simulink model "Aero_Generic"  (R2016b)
settings: Solver=VariableStepAuto  StartTime=0.0  StopTime=10.0  RelTol=1e-3
values from neighbouring files (symbols this model uses):
  AC =     [UAV_modelconfig.mat]
libraries: OpenFlightUtilLib x3
settings Model: Creator=UAVLAB  LastModifiedBy=rega0051

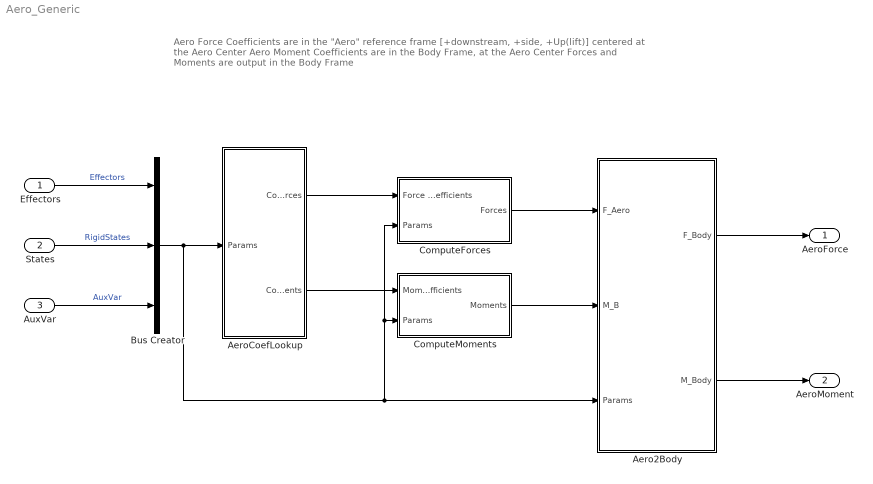
== system Aero_Generic ==
  note: Aero Force Coefficients are in the "Aero" reference frame [+downstream, +side, +Up(lift)] centered at the Aero Center
      | Aero Moment Coefficients are in the Body Frame, at the Aero Center
      |
      | Forces and Moments are output in the Body Frame
  Effectors : Inport  OutDataTypeStr=Bus: Effectors
  States : Inport  Port=2  OutDataTypeStr=Bus: RigidStates
  AuxVar : Inport  Port=3  OutDataTypeStr=Bus: AuxVar
  Aero2Body : Subsystem
  AeroCoefLookup : Subsystem
  Bus Creator : BusCreator  Inputs=3
  ComputeForces : Subsystem
  ComputeMoments : Subsystem
  AeroForce : Outport
  AeroMoment : Outport  Port=2
  wires:
  States/1 -> Bus Creator/2  "RigidStates"
  AuxVar/1 -> Bus Creator/3  "AuxVar"
  Effectors/1 -> Bus Creator/1  "Effectors"
  Bus Creator/1 -> Aero2Body/3(Params), ComputeForces/2(Params), ComputeMoments/2(Params), AeroCoefLookup/1(Params)
  ComputeForces/1(Forces) -> Aero2Body/1(F_Aero)
  ComputeMoments/1(Moments) -> Aero2Body/2(M_B)
  Aero2Body/1(F_Body) -> AeroForce/1
  Aero2Body/2(M_Body) -> AeroMoment/1
  AeroCoefLookup/1(CoefForces) -> ComputeForces/1(Force Coefficients)
  AeroCoefLookup/2(CoefMoments) -> ComputeMoments/1(Moment Coefficients)

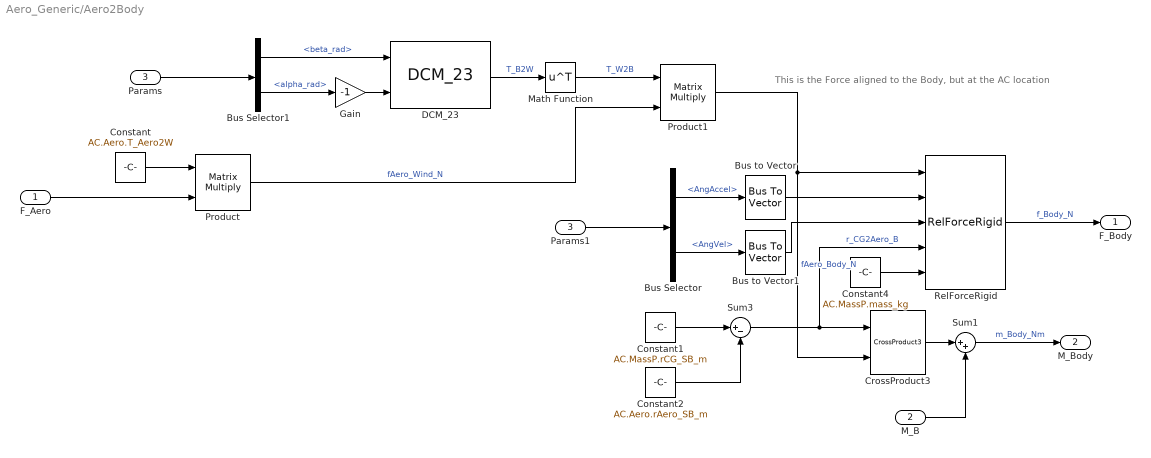
== system Aero_Generic/Aero2Body ==
  note: This is the Force aligned to the Body, but at the AC location
  F_Aero : Inport
  M_B : Inport  Port=2
  Params : Inport  Port=3
  Bus Selector : BusSelector  OutputSignals=RigidStates.AngAccel,RigidStates.AngVel
  Bus Selector1 : BusSelector  OutputSignals=AuxVar.WindAxesParams.beta_rad,AuxVar.WindAxesParams.alpha_rad
  Bus to Vector : BusToVector
  Bus to Vector1 : BusToVector
  Constant : Constant  Value=AC.Aero.T_Aero2W
      settings: AttributesFormatString=%<Value>
  Constant1 : Constant  Value=AC.MassP.rCG_SB_m
      settings: AttributesFormatString=%<Value>
  Constant2 : Constant  Value=AC.Aero.rAero_SB_m
      settings: AttributesFormatString=%<Value>
  Constant4 : Constant  Value=AC.MassP.mass_kg
      settings: AttributesFormatString=%<Value>
  CrossProduct3 : OpenFlightUtilLib/Math/CrossProduct3
  DCM_23 : OpenFlightUtilLib/Transformations/DCM_23
  Gain : Gain  Gain=-1
  Math Function : Math  Operator=transpose  SaturateOnIntegerOverflow=on
  Params1 : InportShadow  Port=3
  Product : Product  Multiplication=Matrix(*)  RndMeth=Zero
  Product1 : Product  Multiplication=Matrix(*)  RndMeth=Zero
  RelForceRigid : OpenFlightUtilLib/Kinematics and Dynamics/RelForceRigid
  Sum1 : Sum  Inputs=|++  SaturateOnIntegerOverflow=on
  Sum3 : Sum  Inputs=|+-  SaturateOnIntegerOverflow=on
  F_Body : Outport
  M_Body : Outport  Port=2
  wires:
  Constant1/1 -> Sum3/1
  Constant2/1 -> Sum3/2
  Bus Selector/1 -> Bus to Vector/1  "<AngAccel>"
  Bus to Vector/1 -> RelForceRigid/2
  Bus to Vector1/1 -> RelForceRigid/3
  Bus Selector/2 -> Bus to Vector1/1  "<AngVel>"
  F_Aero/1 -> Product/2
  Constant/1 -> Product/1
  Params/1 -> Bus Selector1/1
  Math Function/1 -> Product1/1  "T_W2B"
  DCM_23/1 -> Math Function/1  "T_B2W"
  Product/1 -> Product1/2  "fAero_Wind_N"
  Product1/1 -> CrossProduct3/2, RelForceRigid/1  "fAero_Body_N"
  Sum3/1 -> RelForceRigid/4, CrossProduct3/1  "r_CG2Aero_B"
  Params1/1 -> Bus Selector/1
  RelForceRigid/1 -> F_Body/1  "f_Body_N"
  M_B/1 -> Sum1/2
  CrossProduct3/1 -> Sum1/1
  Sum1/1 -> M_Body/1  "m_Body_Nm"
  Constant4/1 -> RelForceRigid/5
  Bus Selector1/1 -> DCM_23/1  "<beta_rad>"
  Bus Selector1/2 -> Gain/1  "<alpha_rad>"
  Gain/1 -> DCM_23/2

== system Aero_Generic/AeroCoefLookup ==
  Params : Inport
  DragCoefficient : Subsystem
  Lift Coefficient : Subsystem
  Mux : Mux  Inputs=3
  Mux1 : Mux  Inputs=3
  PitchMomentCoefficient : Subsystem
  RollMomentCoefficient : Subsystem
  SideForceCoefficient : Subsystem
  YawMomentCoefficient : Subsystem
  CoefForces : Outport
  CoefMoments : Outport  Port=2
  wires:
  Mux1/1 -> CoefMoments/1  "coefMom_B"
  SideForceCoefficient/1(CY) -> Mux/2
  PitchMomentCoefficient/1(Cm) -> Mux1/2
  Mux/1 -> CoefForces/1  "coefF_Aero"
  RollMomentCoefficient/1(Cl) -> Mux1/1
  Lift Coefficient/1(CL) -> DragCoefficient/2(CL), Mux/3
  YawMomentCoefficient/1(Cn) -> Mux1/3
  DragCoefficient/1(CD) -> Mux/1
  Params/1 -> YawMomentCoefficient/1(Params), PitchMomentCoefficient/1(Params), RollMomentCoefficient/1(Params), Lift Coefficient/1(Params), SideForceCoefficient/1(Params), DragCoefficient/1(Params)

== system Aero_Generic/ComputeForces ==
  Force Coefficients : Inport
  Params : Inport  Port=2
  Bus Selector : BusSelector  OutputSignals=AuxVar.qBar_Pa
  Demux3 : Demux  Outputs=3
  Gain2 : Gain  Gain=AC.Geometry.S  SaturateOnIntegerOverflow=on  OutDataTypeStr=Inherit: Same as input  ParamDataTypeStr=Inherit: Same as input
      settings: AttributesFormatString=%<Gain>
  Mux1 : Mux  Inputs=3
  Product6 : Product  SaturateOnIntegerOverflow=on  InputSameDT=on  OutDataTypeStr=Inherit: Same as first input
  Product7 : Product  SaturateOnIntegerOverflow=on  InputSameDT=on  OutDataTypeStr=Inherit: Same as first input
  Product8 : Product  SaturateOnIntegerOverflow=on  InputSameDT=on  OutDataTypeStr=Inherit: Same as first input
  Forces : Outport
  wires:
  Product6/1 -> Mux1/1  "fD_N"
  Product8/1 -> Mux1/3  "fL_N"
  Product7/1 -> Mux1/2  "fY_N"
  Mux1/1 -> Forces/1  "fAero_N"
  Demux3/2 -> Product7/1  "cY"
  Demux3/1 -> Product6/1  "cD"
  Demux3/3 -> Product8/1  "cL"
  Force Coefficients/1 -> Demux3/1
  Gain2/1 -> Product6/2, Product7/2, Product8/2
  Bus Selector/1 -> Gain2/1  "<qBar_Pa>"
  Params/1 -> Bus Selector/1

== system Aero_Generic/ComputeMoments ==
  Moment Coefficients : Inport
  Params : Inport  Port=2
  Bus Selector : BusSelector  OutputSignals=AuxVar.qBar_Pa
  Demux3 : Demux  Outputs=3
  Gain1 : Gain  Gain=AC.Geometry.b  SaturateOnIntegerOverflow=on  OutDataTypeStr=Inherit: Same as input  ParamDataTypeStr=Inherit: Same as input
      settings: AttributesFormatString=%<Gain>
  Gain2 : Gain  Gain=AC.Geometry.S  SaturateOnIntegerOverflow=on  OutDataTypeStr=Inherit: Same as input  ParamDataTypeStr=Inherit: Same as input
      settings: AttributesFormatString=%<Gain>
  Gain3 : Gain  Gain=AC.Geometry.b  SaturateOnIntegerOverflow=on  OutDataTypeStr=Inherit: Same as input  ParamDataTypeStr=Inherit: Same as input
      settings: AttributesFormatString=%<Gain>
  Gain4 : Gain  Gain=AC.Geometry.c  SaturateOnIntegerOverflow=on  OutDataTypeStr=Inherit: Same as input  ParamDataTypeStr=Inherit: Same as input
      settings: AttributesFormatString=%<Gain>
  Mux1 : Mux  Inputs=3
  Product6 : Product  SaturateOnIntegerOverflow=on  InputSameDT=on  OutDataTypeStr=Inherit: Same as first input
  Product7 : Product  SaturateOnIntegerOverflow=on  InputSameDT=on  OutDataTypeStr=Inherit: Same as first input
  Product8 : Product  SaturateOnIntegerOverflow=on  InputSameDT=on  OutDataTypeStr=Inherit: Same as first input
  Moments : Outport
  wires:
  Product6/1 -> Mux1/1  "mL_Nm"
  Product8/1 -> Mux1/3  "mN_Nm"
  Moment Coefficients/1 -> Demux3/1
  Product7/1 -> Mux1/2  "mM_Nm"
  Gain3/1 -> Product8/2
  Mux1/1 -> Moments/1  "mAero_Nm"
  Gain1/1 -> Product6/2
  Gain2/1 -> Gain1/1, Gain4/1, Gain3/1
  Demux3/2 -> Product7/1  "Cm"
  Gain4/1 -> Product7/2
  Demux3/1 -> Product6/1  "Cl"
  Demux3/3 -> Product8/1  "Cn"
  Bus Selector/1 -> Gain2/1  "<qBar_Pa>"
  Params/1 -> Bus Selector/1

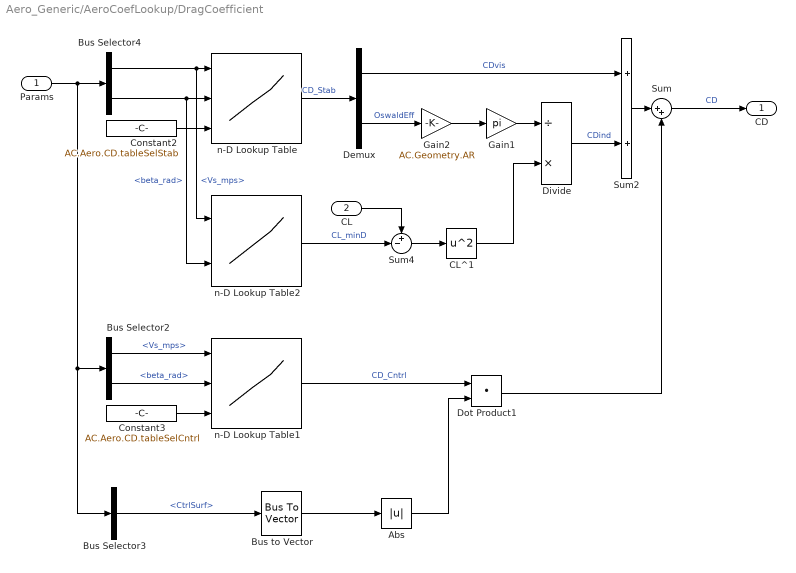
== system Aero_Generic/AeroCoefLookup/DragCoefficient ==
  Params : Inport
  CL : Inport  Port=2
  Abs : Abs
  Bus Selector2 : BusSelector  OutputSignals=AuxVar.WindAxesParams.Vs_mps,AuxVar.WindAxesParams.beta_rad
  Bus Selector3 : BusSelector  OutputSignals=Effectors.CtrlSurf
  Bus Selector4 : BusSelector  OutputSignals=AuxVar.WindAxesParams.Vs_mps,AuxVar.WindAxesParams.beta_rad
  Bus to Vector : BusToVector
  CL^1 : Math  Operator=square  SaturateOnIntegerOverflow=on
  Constant2 : Constant  Value=AC.Aero.CD.tableSelStab
      settings: AttributesFormatString=%<Value>
  Constant3 : Constant  Value=AC.Aero.CD.tableSelCntrl
      settings: AttributesFormatString=%<Value>
  Demux : Demux  Outputs=length(AC.Aero.CD.tableSelStab)
  Divide : Product  Inputs=/*
  Dot Product1 : DotProduct  InputSameDT=on  OutDataTypeStr=Inherit: Inherit via internal rule
  Gain1 : Gain  Gain=pi  SaturateOnIntegerOverflow=on  OutDataTypeStr=Inherit: Same as input  ParamDataTypeStr=Inherit: Same as input
      settings: AttributesFormatString=%<Gain>
  Gain2 : Gain  Gain=AC.Geometry.AR  SaturateOnIntegerOverflow=on  OutDataTypeStr=Inherit: Same as input  ParamDataTypeStr=Inherit: Same as input
      settings: AttributesFormatString=%<Gain>
  Sum : Sum  Inputs=|++
  Sum2 : Sum  SaturateOnIntegerOverflow=on  InputSameDT=on  OutDataTypeStr=Inherit: Same as first input
  Sum4 : Sum  Inputs=+-|  SaturateOnIntegerOverflow=on  InputSameDT=on  OutDataTypeStr=Inherit: Same as first input
  n-D Lookup Table : Lookup_n-D  NumberOfTableDimensions=3  BreakpointsForDimension1=AC.Aero.breakPts{1}  BreakpointsForDimension2=AC.Aero.breakPts{2}  BreakpointsForDimension3=AC.Aero.CD.tableSelStab  Table=AC.Aero.CD.tableStab  InternalRulePriority=Speed  RndMeth=Simplest  InputSameDT=on
      settings: AttributesFormatString=%<Table>
  n-D Lookup Table1 : Lookup_n-D  NumberOfTableDimensions=3  BreakpointsForDimension1=AC.Aero.breakPts{1}  BreakpointsForDimension2=AC.Aero.breakPts{2}  BreakpointsForDimension3=AC.Aero.CD.tableSelCntrl  Table=AC.Aero.CD.tableCntrl  InternalRulePriority=Speed  RndMeth=Simplest  InputSameDT=on
      settings: AttributesFormatString=%<Table>
  n-D Lookup Table2 : Lookup_n-D  BreakpointsForDimension1=AC.Aero.breakPts{1}  BreakpointsForDimension2=AC.Aero.breakPts{2}  BreakpointsForDimension3=AC.Aero.CDw.tableSelStab  Table=AC.Aero.CL.minD  InternalRulePriority=Speed  RndMeth=Simplest  InputSameDT=on
      settings: AttributesFormatString=%<Table>
  CD : Outport
  wires:
  Sum/1 -> CD/1  "CD"
  Sum4/1 -> CL^1/1
  Bus Selector4/2 -> n-D Lookup Table2/2, n-D Lookup Table/2  "<beta_rad>"
  Constant2/1 -> n-D Lookup Table/3
  Bus Selector4/1 -> n-D Lookup Table2/1, n-D Lookup Table/1  "<Vs_mps>"
  n-D Lookup Table/1 -> Demux/1  "CD_Stab"
  Bus Selector3/1 -> Bus to Vector/1  "<CtrlSurf>"
  Bus Selector2/1 -> n-D Lookup Table1/1  "<Vs_mps>"
  Bus Selector2/2 -> n-D Lookup Table1/2  "<beta_rad>"
  Params/1 -> Bus Selector4/1, Bus Selector3/1, Bus Selector2/1
  Constant3/1 -> n-D Lookup Table1/3
  Bus to Vector/1 -> Abs/1
  n-D Lookup Table1/1 -> Dot Product1/1  "CD_Cntrl"
  Dot Product1/1 -> Sum/2
  Demux/1 -> Sum2/1  "CDvis"
  Demux/2 -> Gain2/1  "OswaldEff"
  CL/1 -> Sum4/1
  n-D Lookup Table2/1 -> Sum4/2  "CL_minD"
  Gain2/1 -> Gain1/1
  CL^1/1 -> Divide/2
  Gain1/1 -> Divide/1
  Sum2/1 -> Sum/1
  Divide/1 -> Sum2/2  "CDind"
  Abs/1 -> Dot Product1/2

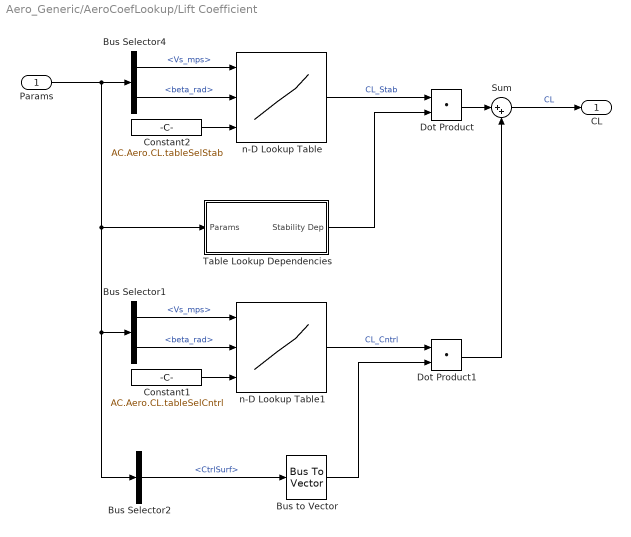
== system Aero_Generic/AeroCoefLookup/Lift Coefficient ==
  Params : Inport
  Bus Selector1 : BusSelector  OutputSignals=AuxVar.WindAxesParams.Vs_mps,AuxVar.WindAxesParams.beta_rad
  Bus Selector2 : BusSelector  OutputSignals=Effectors.CtrlSurf
  Bus Selector4 : BusSelector  OutputSignals=AuxVar.WindAxesParams.Vs_mps,AuxVar.WindAxesParams.beta_rad
  Bus to Vector : BusToVector
  Constant1 : Constant  Value=AC.Aero.CL.tableSelCntrl
      settings: AttributesFormatString=%<Value>
  Constant2 : Constant  Value=AC.Aero.CL.tableSelStab
      settings: AttributesFormatString=%<Value>
  Dot Product : DotProduct  InputSameDT=on  OutDataTypeStr=Inherit: Inherit via internal rule
  Dot Product1 : DotProduct  InputSameDT=on  OutDataTypeStr=Inherit: Inherit via internal rule
  Sum : Sum  Inputs=|++
  Table Lookup Dependencies : Subsystem
  n-D Lookup Table : Lookup_n-D  NumberOfTableDimensions=3  BreakpointsForDimension1=AC.Aero.breakPts{1}  BreakpointsForDimension2=AC.Aero.breakPts{2}  BreakpointsForDimension3=AC.Aero.CL.tableSelStab  Table=AC.Aero.CL.tableStab  InternalRulePriority=Speed  RndMeth=Simplest  InputSameDT=on
      settings: AttributesFormatString=%<Table>
  n-D Lookup Table1 : Lookup_n-D  NumberOfTableDimensions=3  BreakpointsForDimension1=AC.Aero.breakPts{1}  BreakpointsForDimension2=AC.Aero.breakPts{2}  BreakpointsForDimension3=AC.Aero.CL.tableSelCntrl  Table=AC.Aero.CL.tableCntrl  InternalRulePriority=Speed  RndMeth=Simplest  InputSameDT=on
      settings: AttributesFormatString=%<Table>
  CL : Outport
  wires:
  Dot Product/1 -> Sum/1
  Bus Selector4/1 -> n-D Lookup Table/1  "<Vs_mps>"
  Bus Selector4/2 -> n-D Lookup Table/2  "<beta_rad>"
  Constant2/1 -> n-D Lookup Table/3
  n-D Lookup Table/1 -> Dot Product/1  "CL_Stab"
  Bus Selector2/1 -> Bus to Vector/1  "<CtrlSurf>"
  Table Lookup Dependencies/1(Stability Dep) -> Dot Product/2
  Bus Selector1/1 -> n-D Lookup Table1/1  "<Vs_mps>"
  Bus Selector1/2 -> n-D Lookup Table1/2  "<beta_rad>"
  Params/1 -> Bus Selector4/1, Bus Selector2/1, Bus Selector1/1, Table Lookup Dependencies/1(Params)
  Constant1/1 -> n-D Lookup Table1/3
  Bus to Vector/1 -> Dot Product1/2
  n-D Lookup Table1/1 -> Dot Product1/1  "CL_Cntrl"
  Dot Product1/1 -> Sum/2
  Sum/1 -> CL/1  "CL"

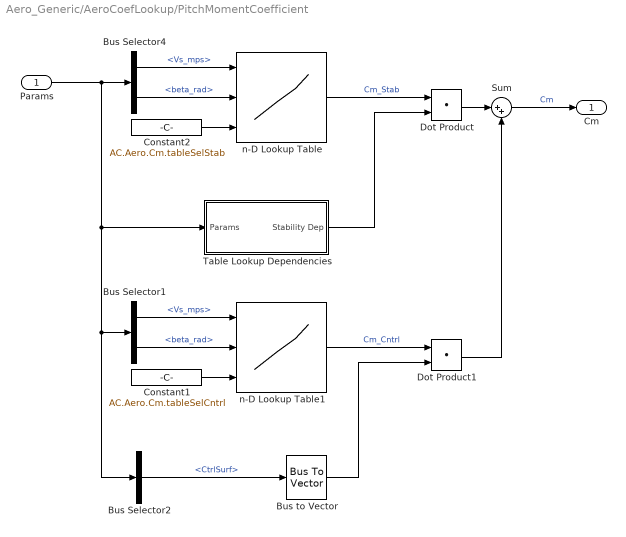
== system Aero_Generic/AeroCoefLookup/PitchMomentCoefficient ==
  Params : Inport
  Bus Selector1 : BusSelector  OutputSignals=AuxVar.WindAxesParams.Vs_mps,AuxVar.WindAxesParams.beta_rad
  Bus Selector2 : BusSelector  OutputSignals=Effectors.CtrlSurf
  Bus Selector4 : BusSelector  OutputSignals=AuxVar.WindAxesParams.Vs_mps,AuxVar.WindAxesParams.beta_rad
  Bus to Vector : BusToVector
  Constant1 : Constant  Value=AC.Aero.Cm.tableSelCntrl
      settings: AttributesFormatString=%<Value>
  Constant2 : Constant  Value=AC.Aero.Cm.tableSelStab
      settings: AttributesFormatString=%<Value>
  Dot Product : DotProduct  InputSameDT=on  OutDataTypeStr=Inherit: Inherit via internal rule
  Dot Product1 : DotProduct  InputSameDT=on  OutDataTypeStr=Inherit: Inherit via internal rule
  Sum : Sum  Inputs=|++
  Table Lookup Dependencies : Subsystem
  n-D Lookup Table : Lookup_n-D  NumberOfTableDimensions=3  BreakpointsForDimension1=AC.Aero.breakPts{1}  BreakpointsForDimension2=AC.Aero.breakPts{2}  BreakpointsForDimension3=AC.Aero.Cm.tableSelStab  Table=AC.Aero.Cm.tableStab  InternalRulePriority=Speed  RndMeth=Simplest  InputSameDT=on
      settings: AttributesFormatString=%<Table>
  n-D Lookup Table1 : Lookup_n-D  NumberOfTableDimensions=3  BreakpointsForDimension1=AC.Aero.breakPts{1}  BreakpointsForDimension2=AC.Aero.breakPts{2}  BreakpointsForDimension3=AC.Aero.Cm.tableSelCntrl  Table=AC.Aero.Cm.tableCntrl  InternalRulePriority=Speed  RndMeth=Simplest  InputSameDT=on
      settings: AttributesFormatString=%<Table>
  Cm : Outport
  wires:
  Dot Product/1 -> Sum/1
  Bus Selector4/1 -> n-D Lookup Table/1  "<Vs_mps>"
  Bus Selector4/2 -> n-D Lookup Table/2  "<beta_rad>"
  Constant2/1 -> n-D Lookup Table/3
  n-D Lookup Table/1 -> Dot Product/1  "Cm_Stab"
  Bus Selector2/1 -> Bus to Vector/1  "<CtrlSurf>"
  Table Lookup Dependencies/1(Stability Dep) -> Dot Product/2
  Bus Selector1/1 -> n-D Lookup Table1/1  "<Vs_mps>"
  Bus Selector1/2 -> n-D Lookup Table1/2  "<beta_rad>"
  Params/1 -> Bus Selector4/1, Bus Selector2/1, Bus Selector1/1, Table Lookup Dependencies/1(Params)
  Constant1/1 -> n-D Lookup Table1/3
  Bus to Vector/1 -> Dot Product1/2
  n-D Lookup Table1/1 -> Dot Product1/1  "Cm_Cntrl"
  Dot Product1/1 -> Sum/2
  Sum/1 -> Cm/1  "Cm"

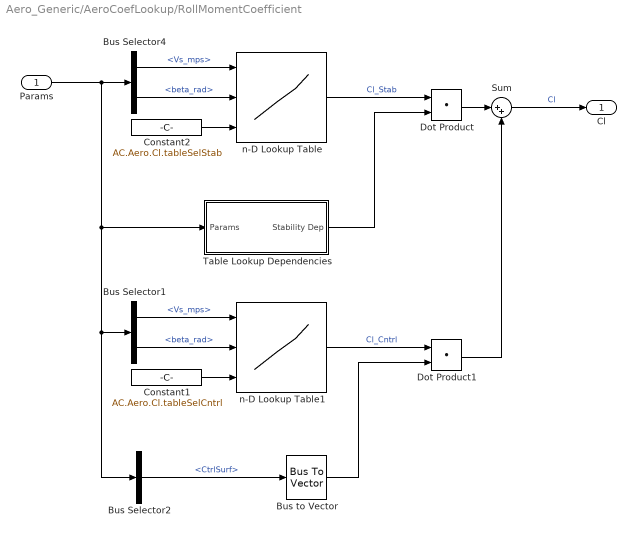
== system Aero_Generic/AeroCoefLookup/RollMomentCoefficient ==
  Params : Inport
  Bus Selector1 : BusSelector  OutputSignals=AuxVar.WindAxesParams.Vs_mps,AuxVar.WindAxesParams.beta_rad
  Bus Selector2 : BusSelector  OutputSignals=Effectors.CtrlSurf
  Bus Selector4 : BusSelector  OutputSignals=AuxVar.WindAxesParams.Vs_mps,AuxVar.WindAxesParams.beta_rad
  Bus to Vector : BusToVector
  Constant1 : Constant  Value=AC.Aero.Cl.tableSelCntrl
      settings: AttributesFormatString=%<Value>
  Constant2 : Constant  Value=AC.Aero.Cl.tableSelStab
      settings: AttributesFormatString=%<Value>
  Dot Product : DotProduct  InputSameDT=on  OutDataTypeStr=Inherit: Inherit via internal rule
  Dot Product1 : DotProduct  InputSameDT=on  OutDataTypeStr=Inherit: Inherit via internal rule
  Sum : Sum  Inputs=|++
  Table Lookup Dependencies : Subsystem
  n-D Lookup Table : Lookup_n-D  NumberOfTableDimensions=3  BreakpointsForDimension1=AC.Aero.breakPts{1}  BreakpointsForDimension2=AC.Aero.breakPts{2}  BreakpointsForDimension3=AC.Aero.Cl.tableSelStab  Table=AC.Aero.Cl.tableStab  InternalRulePriority=Speed  RndMeth=Simplest  InputSameDT=on
      settings: AttributesFormatString=%<Table>
  n-D Lookup Table1 : Lookup_n-D  NumberOfTableDimensions=3  BreakpointsForDimension1=AC.Aero.breakPts{1}  BreakpointsForDimension2=AC.Aero.breakPts{2}  BreakpointsForDimension3=AC.Aero.Cl.tableSelCntrl  Table=AC.Aero.Cl.tableCntrl  InternalRulePriority=Speed  RndMeth=Simplest  InputSameDT=on
      settings: AttributesFormatString=%<Table>
  Cl : Outport
  wires:
  Dot Product/1 -> Sum/1
  Bus Selector4/1 -> n-D Lookup Table/1  "<Vs_mps>"
  Bus Selector4/2 -> n-D Lookup Table/2  "<beta_rad>"
  Constant2/1 -> n-D Lookup Table/3
  n-D Lookup Table/1 -> Dot Product/1  "Cl_Stab"
  Bus Selector2/1 -> Bus to Vector/1  "<CtrlSurf>"
  Table Lookup Dependencies/1(Stability Dep) -> Dot Product/2
  Bus Selector1/1 -> n-D Lookup Table1/1  "<Vs_mps>"
  Bus Selector1/2 -> n-D Lookup Table1/2  "<beta_rad>"
  Params/1 -> Bus Selector4/1, Bus Selector2/1, Bus Selector1/1, Table Lookup Dependencies/1(Params)
  Constant1/1 -> n-D Lookup Table1/3
  Bus to Vector/1 -> Dot Product1/2
  n-D Lookup Table1/1 -> Dot Product1/1  "Cl_Cntrl"
  Dot Product1/1 -> Sum/2
  Sum/1 -> Cl/1  "Cl"

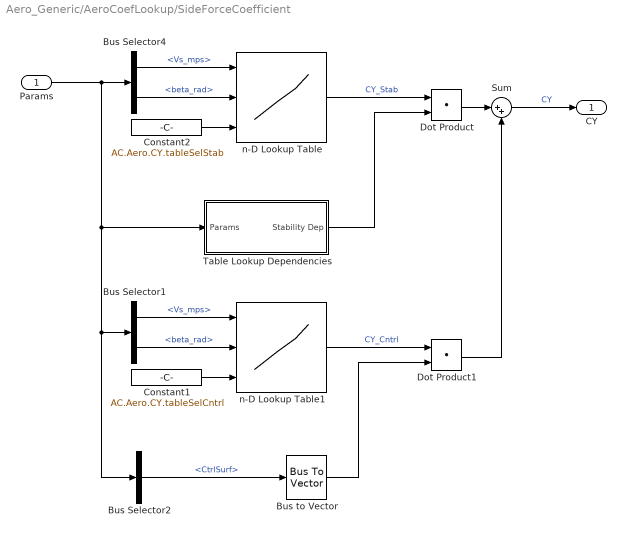
== system Aero_Generic/AeroCoefLookup/SideForceCoefficient ==
  Params : Inport
  Bus Selector1 : BusSelector  OutputSignals=AuxVar.WindAxesParams.Vs_mps,AuxVar.WindAxesParams.beta_rad
  Bus Selector2 : BusSelector  OutputSignals=Effectors.CtrlSurf
  Bus Selector4 : BusSelector  OutputSignals=AuxVar.WindAxesParams.Vs_mps,AuxVar.WindAxesParams.beta_rad
  Bus to Vector : BusToVector
  Constant1 : Constant  Value=AC.Aero.CY.tableSelCntrl
      settings: AttributesFormatString=%<Value>
  Constant2 : Constant  Value=AC.Aero.CY.tableSelStab
      settings: AttributesFormatString=%<Value>
  Dot Product : DotProduct  InputSameDT=on  OutDataTypeStr=Inherit: Inherit via internal rule
  Dot Product1 : DotProduct  InputSameDT=on  OutDataTypeStr=Inherit: Inherit via internal rule
  Sum : Sum  Inputs=|++
  Table Lookup Dependencies : Subsystem
  n-D Lookup Table : Lookup_n-D  NumberOfTableDimensions=3  BreakpointsForDimension1=AC.Aero.breakPts{1}  BreakpointsForDimension2=AC.Aero.breakPts{2}  BreakpointsForDimension3=AC.Aero.CY.tableSelStab  Table=AC.Aero.CY.tableStab  InternalRulePriority=Speed  RndMeth=Simplest  InputSameDT=on
      settings: AttributesFormatString=%<Table>
  n-D Lookup Table1 : Lookup_n-D  NumberOfTableDimensions=3  BreakpointsForDimension1=AC.Aero.breakPts{1}  BreakpointsForDimension2=AC.Aero.breakPts{2}  BreakpointsForDimension3=AC.Aero.CY.tableSelCntrl  Table=AC.Aero.CY.tableCntrl  InternalRulePriority=Speed  RndMeth=Simplest  InputSameDT=on
      settings: AttributesFormatString=%<Table>
  CY : Outport
  wires:
  Dot Product/1 -> Sum/1
  Bus Selector4/1 -> n-D Lookup Table/1  "<Vs_mps>"
  Bus Selector4/2 -> n-D Lookup Table/2  "<beta_rad>"
  Constant2/1 -> n-D Lookup Table/3
  n-D Lookup Table/1 -> Dot Product/1  "CY_Stab"
  Bus Selector2/1 -> Bus to Vector/1  "<CtrlSurf>"
  Table Lookup Dependencies/1(Stability Dep) -> Dot Product/2
  Bus Selector1/1 -> n-D Lookup Table1/1  "<Vs_mps>"
  Bus Selector1/2 -> n-D Lookup Table1/2  "<beta_rad>"
  Params/1 -> Bus Selector4/1, Bus Selector2/1, Bus Selector1/1, Table Lookup Dependencies/1(Params)
  Constant1/1 -> n-D Lookup Table1/3
  Bus to Vector/1 -> Dot Product1/2
  n-D Lookup Table1/1 -> Dot Product1/1  "CY_Cntrl"
  Dot Product1/1 -> Sum/2
  Sum/1 -> CY/1  "CY"

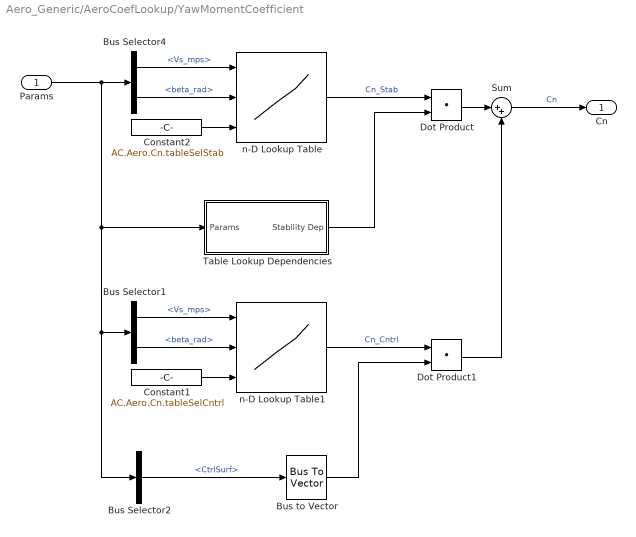
== system Aero_Generic/AeroCoefLookup/YawMomentCoefficient ==
  Params : Inport
  Bus Selector1 : BusSelector  OutputSignals=AuxVar.WindAxesParams.Vs_mps,AuxVar.WindAxesParams.beta_rad
  Bus Selector2 : BusSelector  OutputSignals=Effectors.CtrlSurf
  Bus Selector4 : BusSelector  OutputSignals=AuxVar.WindAxesParams.Vs_mps,AuxVar.WindAxesParams.beta_rad
  Bus to Vector : BusToVector
  Constant1 : Constant  Value=AC.Aero.Cn.tableSelCntrl
      settings: AttributesFormatString=%<Value>
  Constant2 : Constant  Value=AC.Aero.Cn.tableSelStab
      settings: AttributesFormatString=%<Value>
  Dot Product : DotProduct  InputSameDT=on  OutDataTypeStr=Inherit: Inherit via internal rule
  Dot Product1 : DotProduct  InputSameDT=on  OutDataTypeStr=Inherit: Inherit via internal rule
  Sum : Sum  Inputs=|++
  Table Lookup Dependencies : Subsystem
  n-D Lookup Table : Lookup_n-D  NumberOfTableDimensions=3  BreakpointsForDimension1=AC.Aero.breakPts{1}  BreakpointsForDimension2=AC.Aero.breakPts{2}  BreakpointsForDimension3=AC.Aero.Cn.tableSelStab  Table=AC.Aero.Cn.tableStab  InternalRulePriority=Speed  RndMeth=Simplest  InputSameDT=on
      settings: AttributesFormatString=%<Table>
  n-D Lookup Table1 : Lookup_n-D  NumberOfTableDimensions=3  BreakpointsForDimension1=AC.Aero.breakPts{1}  BreakpointsForDimension2=AC.Aero.breakPts{2}  BreakpointsForDimension3=AC.Aero.Cn.tableSelCntrl  Table=AC.Aero.Cn.tableCntrl  InternalRulePriority=Speed  RndMeth=Simplest  InputSameDT=on
      settings: AttributesFormatString=%<Table>
  Cn : Outport
  wires:
  Dot Product/1 -> Sum/1
  Bus Selector4/1 -> n-D Lookup Table/1  "<Vs_mps>"
  Bus Selector4/2 -> n-D Lookup Table/2  "<beta_rad>"
  Constant2/1 -> n-D Lookup Table/3
  n-D Lookup Table/1 -> Dot Product/1  "Cn_Stab"
  Bus Selector2/1 -> Bus to Vector/1  "<CtrlSurf>"
  Table Lookup Dependencies/1(Stability Dep) -> Dot Product/2
  Bus Selector1/1 -> n-D Lookup Table1/1  "<Vs_mps>"
  Bus Selector1/2 -> n-D Lookup Table1/2  "<beta_rad>"
  Params/1 -> Bus Selector4/1, Bus Selector2/1, Bus Selector1/1, Table Lookup Dependencies/1(Params)
  Constant1/1 -> n-D Lookup Table1/3
  Bus to Vector/1 -> Dot Product1/2
  n-D Lookup Table1/1 -> Dot Product1/1  "Cn_Cntrl"
  Dot Product1/1 -> Sum/2
  Sum/1 -> Cn/1  "Cn"

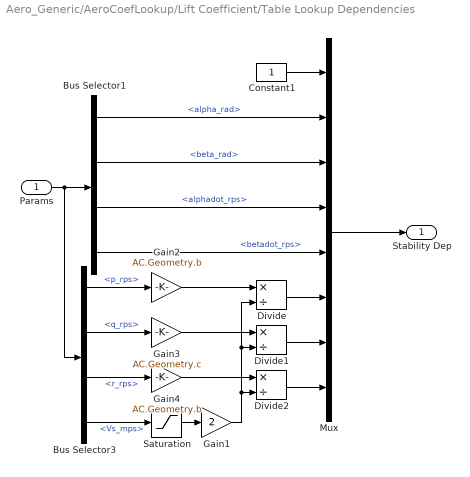
== system Aero_Generic/AeroCoefLookup/Lift Coefficient/Table Lookup Dependencies ==
  Params : Inport
  Bus Selector1 : BusSelector  OutputSignals=AuxVar.WindAxesParams.alpha_rad,AuxVar.WindAxesParams.beta_rad,AuxVar.AlphaBetaDot.alphadot_rps,AuxVar.AlphaBetaDot.betadot_rps
  Bus Selector3 : BusSelector  OutputSignals=RigidStates.AngVel.p_rps,RigidStates.AngVel.q_rps,RigidStates.AngVel.r_rps,AuxVar.WindAxesParams.Vs_mps
  Constant1 : Constant
  Divide : Product  Inputs=*/
  Divide1 : Product  Inputs=*/
  Divide2 : Product  Inputs=*/
  Gain1 : Gain  Gain=2  SaturateOnIntegerOverflow=on  OutDataTypeStr=Inherit: Same as input  ParamDataTypeStr=Inherit: Same as input
  Gain2 : Gain  Gain=AC.Geometry.b  SaturateOnIntegerOverflow=on  OutDataTypeStr=Inherit: Same as input  ParamDataTypeStr=Inherit: Same as input
      settings: AttributesFormatString=%<Gain>
  Gain3 : Gain  Gain=AC.Geometry.c  SaturateOnIntegerOverflow=on  OutDataTypeStr=Inherit: Same as input  ParamDataTypeStr=Inherit: Same as input
      settings: AttributesFormatString=%<Gain>
  Gain4 : Gain  Gain=AC.Geometry.b  SaturateOnIntegerOverflow=on  OutDataTypeStr=Inherit: Same as input  ParamDataTypeStr=Inherit: Same as input
      settings: AttributesFormatString=%<Gain>
  Mux : Mux  Inputs=length(AC.Aero.CL.tableSelStab)
  Saturation : Saturate  UpperLimit=inf  LowerLimit=0.1
  Stability Dep : Outport
  wires:
  Bus Selector1/3 -> Mux/4  "<alphadot_rps>"
  Bus Selector3/4 -> Saturation/1  "<Vs_mps>"
  Divide/1 -> Mux/6
  Bus Selector1/2 -> Mux/3  "<beta_rad>"
  Bus Selector1/4 -> Mux/5  "<betadot_rps>"
  Params/1 -> Bus Selector3/1, Bus Selector1/1
  Constant1/1 -> Mux/1
  Mux/1 -> Stability Dep/1
  Bus Selector1/1 -> Mux/2  "<alpha_rad>"
  Gain2/1 -> Divide/1
  Gain1/1 -> Divide1/2, Divide/2, Divide2/2
  Divide1/1 -> Mux/7
  Divide2/1 -> Mux/8
  Bus Selector3/3 -> Gain4/1  "<r_rps>"
  Gain3/1 -> Divide1/1
  Gain4/1 -> Divide2/1
  Bus Selector3/2 -> Gain3/1  "<q_rps>"
  Bus Selector3/1 -> Gain2/1  "<p_rps>"
  Saturation/1 -> Gain1/1

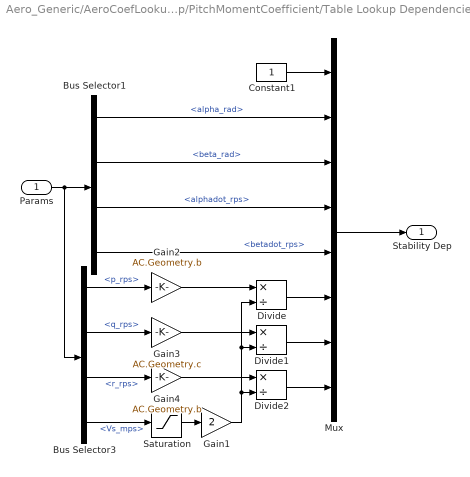
== system Aero_Generic/AeroCoefLookup/PitchMomentCoefficient/Table Lookup Dependencies ==
  Params : Inport
  Bus Selector1 : BusSelector  OutputSignals=AuxVar.WindAxesParams.alpha_rad,AuxVar.WindAxesParams.beta_rad,AuxVar.AlphaBetaDot.alphadot_rps,AuxVar.AlphaBetaDot.betadot_rps
  Bus Selector3 : BusSelector  OutputSignals=RigidStates.AngVel.p_rps,RigidStates.AngVel.q_rps,RigidStates.AngVel.r_rps,AuxVar.WindAxesParams.Vs_mps
  Constant1 : Constant
  Divide : Product  Inputs=*/
  Divide1 : Product  Inputs=*/
  Divide2 : Product  Inputs=*/
  Gain1 : Gain  Gain=2  SaturateOnIntegerOverflow=on  OutDataTypeStr=Inherit: Same as input  ParamDataTypeStr=Inherit: Same as input
  Gain2 : Gain  Gain=AC.Geometry.b  SaturateOnIntegerOverflow=on  OutDataTypeStr=Inherit: Same as input  ParamDataTypeStr=Inherit: Same as input
      settings: AttributesFormatString=%<Gain>
  Gain3 : Gain  Gain=AC.Geometry.c  SaturateOnIntegerOverflow=on  OutDataTypeStr=Inherit: Same as input  ParamDataTypeStr=Inherit: Same as input
      settings: AttributesFormatString=%<Gain>
  Gain4 : Gain  Gain=AC.Geometry.b  SaturateOnIntegerOverflow=on  OutDataTypeStr=Inherit: Same as input  ParamDataTypeStr=Inherit: Same as input
      settings: AttributesFormatString=%<Gain>
  Mux : Mux  Inputs=length(AC.Aero.CL.tableSelStab)
  Saturation : Saturate  UpperLimit=inf  LowerLimit=0.1
  Stability Dep : Outport
  wires:
  Bus Selector1/3 -> Mux/4  "<alphadot_rps>"
  Bus Selector3/4 -> Saturation/1  "<Vs_mps>"
  Divide/1 -> Mux/6
  Bus Selector1/2 -> Mux/3  "<beta_rad>"
  Bus Selector1/4 -> Mux/5  "<betadot_rps>"
  Params/1 -> Bus Selector3/1, Bus Selector1/1
  Constant1/1 -> Mux/1
  Mux/1 -> Stability Dep/1
  Bus Selector1/1 -> Mux/2  "<alpha_rad>"
  Gain2/1 -> Divide/1
  Gain1/1 -> Divide1/2, Divide/2, Divide2/2
  Divide1/1 -> Mux/7
  Divide2/1 -> Mux/8
  Bus Selector3/3 -> Gain4/1  "<r_rps>"
  Gain3/1 -> Divide1/1
  Gain4/1 -> Divide2/1
  Bus Selector3/2 -> Gain3/1  "<q_rps>"
  Bus Selector3/1 -> Gain2/1  "<p_rps>"
  Saturation/1 -> Gain1/1

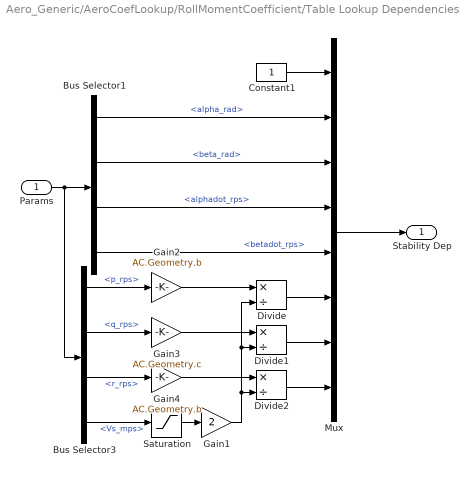
== system Aero_Generic/AeroCoefLookup/RollMomentCoefficient/Table Lookup Dependencies ==
  Params : Inport
  Bus Selector1 : BusSelector  OutputSignals=AuxVar.WindAxesParams.alpha_rad,AuxVar.WindAxesParams.beta_rad,AuxVar.AlphaBetaDot.alphadot_rps,AuxVar.AlphaBetaDot.betadot_rps
  Bus Selector3 : BusSelector  OutputSignals=RigidStates.AngVel.p_rps,RigidStates.AngVel.q_rps,RigidStates.AngVel.r_rps,AuxVar.WindAxesParams.Vs_mps
  Constant1 : Constant
  Divide : Product  Inputs=*/
  Divide1 : Product  Inputs=*/
  Divide2 : Product  Inputs=*/
  Gain1 : Gain  Gain=2  SaturateOnIntegerOverflow=on  OutDataTypeStr=Inherit: Same as input  ParamDataTypeStr=Inherit: Same as input
  Gain2 : Gain  Gain=AC.Geometry.b  SaturateOnIntegerOverflow=on  OutDataTypeStr=Inherit: Same as input  ParamDataTypeStr=Inherit: Same as input
      settings: AttributesFormatString=%<Gain>
  Gain3 : Gain  Gain=AC.Geometry.c  SaturateOnIntegerOverflow=on  OutDataTypeStr=Inherit: Same as input  ParamDataTypeStr=Inherit: Same as input
      settings: AttributesFormatString=%<Gain>
  Gain4 : Gain  Gain=AC.Geometry.b  SaturateOnIntegerOverflow=on  OutDataTypeStr=Inherit: Same as input  ParamDataTypeStr=Inherit: Same as input
      settings: AttributesFormatString=%<Gain>
  Mux : Mux  Inputs=length(AC.Aero.CL.tableSelStab)
  Saturation : Saturate  UpperLimit=inf  LowerLimit=0.1
  Stability Dep : Outport
  wires:
  Bus Selector1/3 -> Mux/4  "<alphadot_rps>"
  Bus Selector3/4 -> Saturation/1  "<Vs_mps>"
  Divide/1 -> Mux/6
  Bus Selector1/2 -> Mux/3  "<beta_rad>"
  Bus Selector1/4 -> Mux/5  "<betadot_rps>"
  Params/1 -> Bus Selector3/1, Bus Selector1/1
  Constant1/1 -> Mux/1
  Mux/1 -> Stability Dep/1
  Bus Selector1/1 -> Mux/2  "<alpha_rad>"
  Gain2/1 -> Divide/1
  Gain1/1 -> Divide1/2, Divide/2, Divide2/2
  Divide1/1 -> Mux/7
  Divide2/1 -> Mux/8
  Bus Selector3/3 -> Gain4/1  "<r_rps>"
  Gain3/1 -> Divide1/1
  Gain4/1 -> Divide2/1
  Bus Selector3/2 -> Gain3/1  "<q_rps>"
  Bus Selector3/1 -> Gain2/1  "<p_rps>"
  Saturation/1 -> Gain1/1

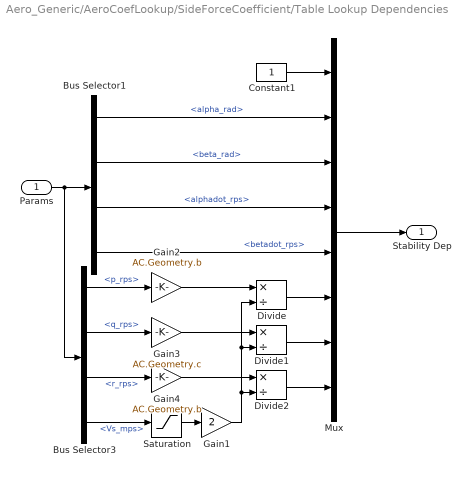
== system Aero_Generic/AeroCoefLookup/SideForceCoefficient/Table Lookup Dependencies ==
  Params : Inport
  Bus Selector1 : BusSelector  OutputSignals=AuxVar.WindAxesParams.alpha_rad,AuxVar.WindAxesParams.beta_rad,AuxVar.AlphaBetaDot.alphadot_rps,AuxVar.AlphaBetaDot.betadot_rps
  Bus Selector3 : BusSelector  OutputSignals=RigidStates.AngVel.p_rps,RigidStates.AngVel.q_rps,RigidStates.AngVel.r_rps,AuxVar.WindAxesParams.Vs_mps
  Constant1 : Constant
  Divide : Product  Inputs=*/
  Divide1 : Product  Inputs=*/
  Divide2 : Product  Inputs=*/
  Gain1 : Gain  Gain=2  SaturateOnIntegerOverflow=on  OutDataTypeStr=Inherit: Same as input  ParamDataTypeStr=Inherit: Same as input
  Gain2 : Gain  Gain=AC.Geometry.b  SaturateOnIntegerOverflow=on  OutDataTypeStr=Inherit: Same as input  ParamDataTypeStr=Inherit: Same as input
      settings: AttributesFormatString=%<Gain>
  Gain3 : Gain  Gain=AC.Geometry.c  SaturateOnIntegerOverflow=on  OutDataTypeStr=Inherit: Same as input  ParamDataTypeStr=Inherit: Same as input
      settings: AttributesFormatString=%<Gain>
  Gain4 : Gain  Gain=AC.Geometry.b  SaturateOnIntegerOverflow=on  OutDataTypeStr=Inherit: Same as input  ParamDataTypeStr=Inherit: Same as input
      settings: AttributesFormatString=%<Gain>
  Mux : Mux  Inputs=length(AC.Aero.CL.tableSelStab)
  Saturation : Saturate  UpperLimit=inf  LowerLimit=0.1
  Stability Dep : Outport
  wires:
  Bus Selector1/3 -> Mux/4  "<alphadot_rps>"
  Bus Selector3/4 -> Saturation/1  "<Vs_mps>"
  Divide/1 -> Mux/6
  Bus Selector1/2 -> Mux/3  "<beta_rad>"
  Bus Selector1/4 -> Mux/5  "<betadot_rps>"
  Params/1 -> Bus Selector3/1, Bus Selector1/1
  Constant1/1 -> Mux/1
  Mux/1 -> Stability Dep/1
  Bus Selector1/1 -> Mux/2  "<alpha_rad>"
  Gain2/1 -> Divide/1
  Gain1/1 -> Divide1/2, Divide/2, Divide2/2
  Divide1/1 -> Mux/7
  Divide2/1 -> Mux/8
  Bus Selector3/3 -> Gain4/1  "<r_rps>"
  Gain3/1 -> Divide1/1
  Gain4/1 -> Divide2/1
  Bus Selector3/2 -> Gain3/1  "<q_rps>"
  Bus Selector3/1 -> Gain2/1  "<p_rps>"
  Saturation/1 -> Gain1/1

== system Aero_Generic/AeroCoefLookup/YawMomentCoefficient/Table Lookup Dependencies ==
  Params : Inport
  Bus Selector1 : BusSelector  OutputSignals=AuxVar.WindAxesParams.alpha_rad,AuxVar.WindAxesParams.beta_rad,AuxVar.AlphaBetaDot.alphadot_rps,AuxVar.AlphaBetaDot.betadot_rps
  Bus Selector3 : BusSelector  OutputSignals=RigidStates.AngVel.p_rps,RigidStates.AngVel.q_rps,RigidStates.AngVel.r_rps,AuxVar.WindAxesParams.Vs_mps
  Constant1 : Constant
  Divide : Product  Inputs=*/
  Divide1 : Product  Inputs=*/
  Divide2 : Product  Inputs=*/
  Gain1 : Gain  Gain=2  SaturateOnIntegerOverflow=on  OutDataTypeStr=Inherit: Same as input  ParamDataTypeStr=Inherit: Same as input
  Gain2 : Gain  Gain=AC.Geometry.b  SaturateOnIntegerOverflow=on  OutDataTypeStr=Inherit: Same as input  ParamDataTypeStr=Inherit: Same as input
      settings: AttributesFormatString=%<Gain>
  Gain3 : Gain  Gain=AC.Geometry.c  SaturateOnIntegerOverflow=on  OutDataTypeStr=Inherit: Same as input  ParamDataTypeStr=Inherit: Same as input
      settings: AttributesFormatString=%<Gain>
  Gain4 : Gain  Gain=AC.Geometry.b  SaturateOnIntegerOverflow=on  OutDataTypeStr=Inherit: Same as input  ParamDataTypeStr=Inherit: Same as input
      settings: AttributesFormatString=%<Gain>
  Mux : Mux  Inputs=length(AC.Aero.CL.tableSelStab)
  Saturation : Saturate  UpperLimit=inf  LowerLimit=0.1
  Stability Dep : Outport
  wires:
  Bus Selector1/3 -> Mux/4  "<alphadot_rps>"
  Bus Selector3/4 -> Saturation/1  "<Vs_mps>"
  Divide/1 -> Mux/6
  Bus Selector1/2 -> Mux/3  "<beta_rad>"
  Bus Selector1/4 -> Mux/5  "<betadot_rps>"
  Params/1 -> Bus Selector3/1, Bus Selector1/1
  Constant1/1 -> Mux/1
  Mux/1 -> Stability Dep/1
  Bus Selector1/1 -> Mux/2  "<alpha_rad>"
  Gain2/1 -> Divide/1
  Gain1/1 -> Divide1/2, Divide/2, Divide2/2
  Divide1/1 -> Mux/7
  Divide2/1 -> Mux/8
  Bus Selector3/3 -> Gain4/1  "<r_rps>"
  Gain3/1 -> Divide1/1
  Gain4/1 -> Divide2/1
  Bus Selector3/2 -> Gain3/1  "<q_rps>"
  Bus Selector3/1 -> Gain2/1  "<p_rps>"
  Saturation/1 -> Gain1/1
